simulink model "D_vs_tdc"  (R2018b)
settings: Solver=ode23t  StartTime=0.0  StopTime=model_time  FixedStep=0.0000001  RelTol=1e-3
values from neighbouring files (symbols this model uses):
  config_lambda = [lambda0 lambdainf lambda0l mu v_z]    [vs_ifac_setup_v2.m]
  h = [1 0]'    [setup_compensator_test.m]    (also in vs_ifac_setup_v2.m = 0.003)
  Kp = diag([4   4   4 4 30])    [vs_ifac_setup_v2.m]
  Kv = diag([2    2   2 2 20])    [vs_ifac_setup_v2.m]
  L = 0.003    [vs_ifac_setup_v2.m]
  p0 = cam.plot(P, 'pose', T)    [vs_ifac_setup_v2.m]
  p_des = [412 412 612 612; 412 612 612 412]    [vs_ifac_setup_v2.m]
  q0 = -[3.3, 1.2, -1, 1.75, 6]'    [vs_ifac_setup_v2.m]
undefined symbols (not defined in the file or in its folder): addMass, DiscIntNeverNeededParam, Dnaw, Kaw, Ki, Upaw, variation
libraries: roblocks x15, simulink x1
(part 3 of 3)

== matlab function D_vs_tdc/ARM Plant (MCG)1/C  ==
  data: q input; dq input; tau output
function tau = getC(q, dq)
G3 = 0;

th1 = q(1);
th2 = q(2);
th3 = q(3);
th4 = q(4);
th5 = q(5);

QP1 = dq(1);
QP2 = dq(2);
QP3 = dq(3);
QP4 = dq(4);
QP5 = dq(5);


XX1 = 0;
XY1 = 0;
XZ1 = 0;
YY1 = 0;
YZ1 = 0;
ZZ1 = 0.7569 * 1.0e-04;
MX1 = 0.0165*0.1390;
MY1 = 0;
MZ1 = -0.0300*0.1390;
M1 = 0.1390;
IA1 = 1.3910e-04;

XX2 = 0.0003;
XY2 = 0;
XZ2 = 0;
YY2 = 0.0106;
YZ2 = 0;
ZZ2 = 0.0106;
MX2 = 0.0775*1.3180;
MY2 = 0;
MZ2 = 0;
M2 = 1.3180;
IA2 = 1.3910e-04;

XX3 = 0.0002;
XY3 = 0;
XZ3 = 0;
YY3 = 0.0050;
YZ3 = 0;
ZZ3 = 0.0050;
MX3 = 0.0675*0.8210;
MY3 = 0;
MZ3 = 0;
M3 = 0.8210;
IA3 = 1.3570e-04;

XX4 = 0.0033;
XY4 = 0;
XZ4 = 0;
YY4 = 0.0002;
YZ4 = 0;
ZZ4 = 0.0033;
MX4 = 0;
MY4 = 0.0568*0.7690;
MZ4 = 0;
M4 = 0.7690;
IA4 = 9.3200e-05;

XX5 = 0;
XY5 = 0;
XZ5 = 0;
YY5 = 0;
YZ5 = 0;
ZZ5 = 0.1820 * 1.0e-04;
MX5 = 0;
MY5 = 0;
MZ5 = 0.*0.0910;
M5 = 0.0910;
IA5 = 3.5700e-05;


% Motors parameters
% FS1 = 0.2;
% FV1 = 0.0012;
% FS2 = 0.2;
% FV2 = 0.0012;
% FS3 = 0.2;
% FV3 = 0.0012;
% FS4 = 0.2;
% FV4 =  0.0012;
% FS5 =  0.2;
% FV5 = 0.0012;
% MZ3 = 0.2;

FS1 = 0;
FV1 = 0.0012;
FS2 = 0;
FV2 = 0.0012;
FS3 = 0;
FV3 = 0.0012;
FS4 = 0;
FV4 =  0.0012;
FS5 =  0;
FV5 = 0.0012;



C_th1 = cos(th1 - 2.9496);
S_th1 = sin(th1 - 2.9496);
C_th2 = cos(th2 - 2.7053);
S_th2 = sin(th2 - 2.7053);
S_th3 = sin(th3 + 2.6354);
C_th3 = cos(th3 + 2.6354);
C_th4 = cos(th4 - 3.3598);
S_th4 = sin(th4 - 3.3598);
S_th5 = sin(th5 - 2.8798);
C_th5 = cos(th5 - 2.8798);
DV61 = QP1^2;
W12 = -QP1*S_th2;
W22 = C_th2*QP1;
WP12 = QP2*W22;
WP22 = -QP2*W12;
DV12 = W12^2;
DV22 = W12*W22;
DV42 = W22^2;
DV62 = QP2^2;
U112 = -DV42 - DV62;
U312 = -2*WP22;
U222 = -DV12 - DV62;
U322 = 2*WP12;
U332 = -DV12 - DV42;
VSP12 = -0.033*DV61;
VP12 = C_th2*VSP12 + G3*S_th2;
VP22 = -C_th2*G3 + S_th2*VSP12;
W13 = C_th3*W12 - S_th3*W22;
W23 = C_th3*W22 + S_th3*W12;
W33 = QP2 + QP3;
WP13 = C_th3*WP12 + QP3*W23 - S_th3*WP22;
WP23 = C_th3*WP22 - QP3*W13 + S_th3*WP12;
DV13 = W13^2;
DV23 = W13*W23;
DV33 = W13*W33;
DV43 = W23^2;
DV53 = W23*W33;
DV63 = W33^2;
U113 = -DV43 - DV63;
U313 = DV33 - WP23;
U223 = -DV13 - DV63;
U323 = DV53 + WP13;
U133 = DV33 + WP23;
U233 = DV53 - WP13;
U333 = -DV13 - DV43;
VSP13 = 0.155*U112 + VP12;
VSP23 = 0.155*DV22 + VP22;
VSP33 = 0.155*U312;
VP13 = C_th3*VSP13 - S_th3*VSP23;
VP23 = C_th3*VSP23 + S_th3*VSP13;
W14 = C_th4*W13 - S_th4*W23;
W24 = C_th4*W23 + S_th4*W13;
W34 = QP4 + W33;
WP14 = C_th4*WP13 + QP4*W24 - S_th4*WP23;
WP24 = C_th4*WP23 - QP4*W14 + S_th4*WP13;
DV14 = W14^2;
DV24 = W14*W24;
DV34 = W14*W34;
DV44 = W24^2;
DV54 = W24*W34;
DV64 = W34^2;
U114 = -DV44 - DV64;
U314 = DV34 - WP24;
U224 = -DV14 - DV64;
U324 = DV54 + WP14;
U134 = DV34 + WP24;
U234 = DV54 - WP14;
U334 = -DV14 - DV44;
VSP14 = 0.135*U113 + VP13;
VSP24 = 0.135*DV23 + VP23;
VSP34 = 0.135*U313 + VSP33;
VP14 = C_th4*VSP14 - S_th4*VSP24;
VP24 = C_th4*VSP24 + S_th4*VSP14;
W15 = C_th5*W14 - S_th5*W34;
W25 = C_th5*W34 + S_th5*W14;
W35 = QP5 - W24;
WP15 = C_th5*WP14 + QP5*W25;
WP25 = -QP5*W15 + S_th5*WP14;
DV15 = W15^2;
DV25 = W15*W25;
DV35 = W15*W35;
DV45 = W25^2;
DV55 = W25*W35;
DV65 = W35^2;
U115 = -DV45 - DV65;
U215 = DV25 - WP24;
U315 = DV35 - WP25;
U125 = DV25 + WP24;
U225 = -DV15 - DV65;
U325 = DV55 + WP15;
U135 = DV35 + WP25;
U235 = DV55 - WP15;
U335 = -DV15 - DV45;
VSP15 = -0.218*DV24 + VP14;
VSP25 = -0.218*U224 + VP24;
VSP35 = -0.218*U324 + VSP34;
VP15 = C_th5*VSP15 - S_th5*VSP35;
VP25 = C_th5*VSP35 + S_th5*VSP15;
F11 = -DV61*MX1;
F21 = -DV61*MY1;
F31 = -G3*M1;
PSI11 = QP1*XZ1;
PSI21 = QP1*YZ1;
PSI31 = QP1*ZZ1;
No11 = -PSI21*QP1;
No21 = PSI11*QP1;
F12 = DV22*MY2 + M2*VP12 + MX2*U112;
F22 = DV22*MX2 + M2*VP22 + MY2*U222;
F32 = MX2*U312 + MY2*U322 + MZ2*U332;
PSI12 = QP2*XZ2 + W12*XX2 + W22*XY2;
PSI22 = QP2*YZ2 + W12*XY2 + W22*YY2;
PSI32 = QP2*ZZ2 + W12*XZ2 + W22*YZ2;
No12 = -PSI22*QP2 + PSI32*W22 + WP12*XX2 + WP22*XY2;
No22 = PSI12*QP2 - PSI32*W12 + WP12*XY2 + WP22*YY2;
No32 = -PSI12*W22 + PSI22*W12 + WP12*XZ2 + WP22*YZ2;
F13 = DV23*MY3 + M3*VP13 + MX3*U113 + MZ3*U133;
F23 = DV23*MX3 + M3*VP23 + MY3*U223 + MZ3*U233;
F33 = M3*VSP33 + MX3*U313 + MY3*U323 + MZ3*U333;
PSI13 = W13*XX3 + W23*XY3 + W33*XZ3;
PSI23 = W13*XY3 + W23*YY3 + W33*YZ3;
PSI33 = W13*XZ3 + W23*YZ3 + W33*ZZ3;
No13 = -PSI23*W33 + PSI33*W23 + WP13*XX3 + WP23*XY3;
No23 = PSI13*W33 - PSI33*W13 + WP13*XY3 + WP23*YY3;
No33 = -PSI13*W23 + PSI23*W13 + WP13*XZ3 + WP23*YZ3;
F14 = DV24*MY4 + M4*VP14 + MX4*U114 + MZ4*U134;
F24 = DV24*MX4 + M4*VP24 + MY4*U224 + MZ4*U234;
F34 = M4*VSP34 + MX4*U314 + MY4*U324 + MZ4*U334;
PSI14 = W14*XX4 + W24*XY4 + W34*XZ4;
PSI24 = W14*XY4 + W24*YY4 + W34*YZ4;
PSI34 = W14*XZ4 + W24*YZ4 + W34*ZZ4;
No14 = -PSI24*W34 + PSI34*W24 + WP14*XX4 + WP24*XY4;
No24 = PSI14*W34 - PSI34*W14 + WP14*XY4 + WP24*YY4;
No34 = -PSI14*W24 + PSI24*W14 + WP14*XZ4 + WP24*YZ4;
F15 = M5*VP15 + MX5*U115 + MY5*U125 + MZ5*U135;
F25 = M5*VP25 + MX5*U215 + MY5*U225 + MZ5*U235;
F35 = -M5*VSP25 + MX5*U315 + MY5*U325 + MZ5*U335;
PSI15 = W15*XX5 + W25*XY5 + W35*XZ5;
PSI25 = W15*XY5 + W25*YY5 + W35*YZ5;
PSI35 = W15*XZ5 + W25*YZ5 + W35*ZZ5;
No15 = -PSI25*W35 + PSI35*W25 + WP15*XX5 - WP24*XZ5 + WP25*XY5;
No25 = PSI15*W35 - PSI35*W15 + WP15*XY5 - WP24*YZ5 + WP25*YY5;
No35 = -PSI15*W25 + PSI25*W15 + WP15*XZ5 - WP24*ZZ5 + WP25*YZ5;
N15 = -MY5*VSP25 - MZ5*VP25 + No15;
N25 = MX5*VSP25 + MZ5*VP15 + No25;
N35 = MX5*VP25 - MY5*VP15 + No35;
FDI15 = C_th5*F15 + F25*S_th5;
FDI35 = C_th5*F25 - F15*S_th5;
E14 = F14 + FDI15;
E24 = F24 - F35;
E34 = F34 + FDI35;
N14 = C_th5*N15 - 0.218*FDI35 + MY4*VSP34 - MZ4*VP24 + N25*S_th5 + No14;
N24 = -MX4*VSP34 + MZ4*VP14 - N35 + No24;
N34 = C_th5*N25 + 0.218*FDI15 + MX4*VP24 - MY4*VP14 - N15*S_th5 + No34;
FDI14 = C_th4*E14 + E24*S_th4;
FDI24 = C_th4*E24 - E14*S_th4;
E13 = F13 + FDI14;
E23 = F23 + FDI24;
E33 = E34 + F33;
N13 = C_th4*N14 + MY3*VSP33 - MZ3*VP23 + N24*S_th4 + No13;
N23 = C_th4*N24 - 0.135*E34 - MX3*VSP33 + MZ3*VP13 - N14*S_th4 + No23;
N33 = 0.135*FDI24 + MX3*VP23 - MY3*VP13 + N34 + No33;
FDI13 = C_th3*E13 + E23*S_th3;
FDI23 = C_th3*E23 - E13*S_th3;
E12 = F12 + FDI13;
E22 = F22 + FDI23;
E32 = E33 + F32;
N12 = C_th3*N13 - MZ2*VP22 + N23*S_th3 + No12;
N22 = C_th3*N23 - 0.155*E33 + MZ2*VP12 - N13*S_th3 + No22;
N32 = 0.155*FDI23 + MX2*VP22 - MY2*VP12 + N33 + No32;
FDI12 = C_th2*E12 + E22*S_th2;
FDI32 = C_th2*E22 - E12*S_th2;
E11 = F11 + FDI12;
E21 = -E32 + F21;
E31 = F31 + FDI32;
N11 = C_th2*N12 - G3*MY1 + N22*S_th2 + No11;
N21 = -0.033*FDI32 + G3*MX1 - N32 + No21;
N31 = C_th2*N22 - 0.033*E32 - N12*S_th2;
FDI11 = C_th1*E11 + E21*S_th1;
FDI21 = C_th1*E21 - E11*S_th1;
GAM1 = FS1*sign(QP1) + FV1*QP1 + N31;
GAM2 = FS2*sign(QP2) + FV2*QP2 + N32;
GAM3 = FS3*sign(QP3) + FV3*QP3 + N33;
GAM4 = FS4*sign(QP4) + FV4*QP4 + N34;
GAM5 = FS5*sign(QP5) + FV5*QP5 + N35;

tau = [GAM1 GAM2 GAM3 GAM4 GAM5]';

== matlab function D_vs_tdc/MCG (Symoro, DD)/C  ==
  data: q input; dq input; tau output
function tau = getC(q, dq)
G3 = -9.81;

th1 = q(1);
th2 = q(2);
th3 = q(3);
th4 = q(4);
th5 = q(5);

QP1 = dq(1);
QP2 = dq(2);
QP3 = dq(3);
QP4 = dq(4);
QP5 = dq(5);


XX1 = 0;
XY1 = 0;
XZ1 = 0;
YY1 = 0;
YZ1 = 0;
ZZ1 = 0.7569 * 1.0e-04;
MX1 = 0.0165*0.1390;
MY1 = 0;
MZ1 = -0.0300;
M1 = 0.1390;
IA1 = 1.3910e-04;

XX2 = 0.0003;
XY2 = 0;
XZ2 = 0;
YY2 = 0.0106;
YZ2 = 0;
ZZ2 = 0.0106;
MX2 = 0.0775*1.3180;
MY2 = 0;
MZ2 = 0;
M2 = 1.3180;
IA2 = 1.3910e-04;

XX3 = 0.0002;
XY3 = 0;
XZ3 = 0;
YY3 = 0.0050;
YZ3 = 0;
ZZ3 = 0.0050;
MX3 = 0.0675*0.8210;
MY3 = 0;
MZ3 = 0;
M3 = 0.8210;
IA3 = 1.3570e-04;

XX4 = 0.0033;
XY4 = 0;
XZ4 = 0;
YY4 = 0.0002;
YZ4 = 0;
ZZ4 = 0.0033;
MX4 = 0;
MY4 = 0.0568*0.7690;
MZ4 = 0;
M4 = 0.7690;
IA4 = 9.3200e-05;

XX5 = 0;
XY5 = 0;
XZ5 = 0;
YY5 = 0;
YZ5 = 0;
ZZ5 = 0.1820 * 1.0e-04;
MX5 = 0;
MY5 = 0;
MZ5 = 0.*0.0910;
M5 = 0.0910;
IA5 = 3.5700e-05;


% Motors parameters
FS1 = 0;
FV1 = 0.0012;
FS2 = 0;
FV2 = 0.0012;
FS3 = 0;
FV3 = 0.0012;
FS4 = 0;
FV4 =  0.0012;
FS5 = 0;
FV5 = 0.0012;

% FS1 = 0;
% FV1 = 0;
% FS2 = 0;
% FV2 = 0;
% FS3 = 0;
% FV3 = 0;
% FS4 = 0;
% FV4 = 0;
% FS5 = 0;
% FV5 = 0;


C_th1 = cos(th1 - 2.9496);
S_th1 = sin(th1 - 2.9496);
C_th2 = cos(th2 - 2.7053);
S_th2 = sin(th2 - 2.7053);
S_th3 = sin(th3 + 2.6354);
C_th3 = cos(th3 + 2.6354);
C_th4 = cos(th4 - 3.3598);
S_th4 = sin(th4 - 3.3598);
S_th5 = sin(th5 - 2.8798);
C_th5 = cos(th5 - 2.8798);
DV61 = QP1^2;
W12 = -QP1*S_th2;
W22 = C_th2*QP1;
WP12 = QP2*W22;
WP22 = -QP2*W12;
DV12 = W12^2;
DV22 = W12*W22;
DV42 = W22^2;
DV62 = QP2^2;
U112 = -DV42 - DV62;
U312 = -2*WP22;
U222 = -DV12 - DV62;
U322 = 2*WP12;
U332 = -DV12 - DV42;
VSP12 = -0.033*DV61;
VP12 = C_th2*VSP12 + G3*S_th2;
VP22 = -C_th2*G3 + S_th2*VSP12;
W13 = C_th3*W12 - S_th3*W22;
W23 = C_th3*W22 + S_th3*W12;
W33 = QP2 + QP3;
WP13 = C_th3*WP12 + QP3*W23 - S_th3*WP22;
WP23 = C_th3*WP22 - QP3*W13 + S_th3*WP12;
DV13 = W13^2;
DV23 = W13*W23;
DV33 = W13*W33;
DV43 = W23^2;
DV53 = W23*W33;
DV63 = W33^2;
U113 = -DV43 - DV63;
U313 = DV33 - WP23;
U223 = -DV13 - DV63;
U323 = DV53 + WP13;
U133 = DV33 + WP23;
U233 = DV53 - WP13;
U333 = -DV13 - DV43;
VSP13 = 0.155*U112 + VP12;
VSP23 = 0.155*DV22 + VP22;
VSP33 = 0.155*U312;
VP13 = C_th3*VSP13 - S_th3*VSP23;
VP23 = C_th3*VSP23 + S_th3*VSP13;
W14 = C_th4*W13 - S_th4*W23;
W24 = C_th4*W23 + S_th4*W13;
W34 = QP4 + W33;
WP14 = C_th4*WP13 + QP4*W24 - S_th4*WP23;
WP24 = C_th4*WP23 - QP4*W14 + S_th4*WP13;
DV14 = W14^2;
DV24 = W14*W24;
DV34 = W14*W34;
DV44 = W24^2;
DV54 = W24*W34;
DV64 = W34^2;
U114 = -DV44 - DV64;
U314 = DV34 - WP24;
U224 = -DV14 - DV64;
U324 = DV54 + WP14;
U134 = DV34 + WP24;
U234 = DV54 - WP14;
U334 = -DV14 - DV44;
VSP14 = 0.135*U113 + VP13;
VSP24 = 0.135*DV23 + VP23;
VSP34 = 0.135*U313 + VSP33;
VP14 = C_th4*VSP14 - S_th4*VSP24;
VP24 = C_th4*VSP24 + S_th4*VSP14;
W15 = C_th5*W14 - S_th5*W34;
W25 = C_th5*W34 + S_th5*W14;
W35 = QP5 - W24;
WP15 = C_th5*WP14 + QP5*W25;
WP25 = -QP5*W15 + S_th5*WP14;
DV15 = W15^2;
DV25 = W15*W25;
DV35 = W15*W35;
DV45 = W25^2;
DV55 = W25*W35;
DV65 = W35^2;
U115 = -DV45 - DV65;
U215 = DV25 - WP24;
U315 = DV35 - WP25;
U125 = DV25 + WP24;
U225 = -DV15 - DV65;
U325 = DV55 + WP15;
U135 = DV35 + WP25;
U235 = DV55 - WP15;
U335 = -DV15 - DV45;
VSP15 = -0.218*DV24 + VP14;
VSP25 = -0.218*U224 + VP24;
VSP35 = -0.218*U324 + VSP34;
VP15 = C_th5*VSP15 - S_th5*VSP35;
VP25 = C_th5*VSP35 + S_th5*VSP15;
F11 = -DV61*MX1;
F21 = -DV61*MY1;
F31 = -G3*M1;
PSI11 = QP1*XZ1;
PSI21 = QP1*YZ1;
PSI31 = QP1*ZZ1;
No11 = -PSI21*QP1;
No21 = PSI11*QP1;
F12 = DV22*MY2 + M2*VP12 + MX2*U112;
F22 = DV22*MX2 + M2*VP22 + MY2*U222;
F32 = MX2*U312 + MY2*U322 + MZ2*U332;
PSI12 = QP2*XZ2 + W12*XX2 + W22*XY2;
PSI22 = QP2*YZ2 + W12*XY2 + W22*YY2;
PSI32 = QP2*ZZ2 + W12*XZ2 + W22*YZ2;
No12 = -PSI22*QP2 + PSI32*W22 + WP12*XX2 + WP22*XY2;
No22 = PSI12*QP2 - PSI32*W12 + WP12*XY2 + WP22*YY2;
No32 = -PSI12*W22 + PSI22*W12 + WP12*XZ2 + WP22*YZ2;
F13 = DV23*MY3 + M3*VP13 + MX3*U113 + MZ3*U133;
F23 = DV23*MX3 + M3*VP23 + MY3*U223 + MZ3*U233;
F33 = M3*VSP33 + MX3*U313 + MY3*U323 + MZ3*U333;
PSI13 = W13*XX3 + W23*XY3 + W33*XZ3;
PSI23 = W13*XY3 + W23*YY3 + W33*YZ3;
PSI33 = W13*XZ3 + W23*YZ3 + W33*ZZ3;
No13 = -PSI23*W33 + PSI33*W23 + WP13*XX3 + WP23*XY3;
No23 = PSI13*W33 - PSI33*W13 + WP13*XY3 + WP23*YY3;
No33 = -PSI13*W23 + PSI23*W13 + WP13*XZ3 + WP23*YZ3;
F14 = DV24*MY4 + M4*VP14 + MX4*U114 + MZ4*U134;
F24 = DV24*MX4 + M4*VP24 + MY4*U224 + MZ4*U234;
F34 = M4*VSP34 + MX4*U314 + MY4*U324 + MZ4*U334;
PSI14 = W14*XX4 + W24*XY4 + W34*XZ4;
PSI24 = W14*XY4 + W24*YY4 + W34*YZ4;
PSI34 = W14*XZ4 + W24*YZ4 + W34*ZZ4;
No14 = -PSI24*W34 + PSI34*W24 + WP14*XX4 + WP24*XY4;
No24 = PSI14*W34 - PSI34*W14 + WP14*XY4 + WP24*YY4;
No34 = -PSI14*W24 + PSI24*W14 + WP14*XZ4 + WP24*YZ4;
F15 = M5*VP15 + MX5*U115 + MY5*U125 + MZ5*U135;
F25 = M5*VP25 + MX5*U215 + MY5*U225 + MZ5*U235;
F35 = -M5*VSP25 + MX5*U315 + MY5*U325 + MZ5*U335;
PSI15 = W15*XX5 + W25*XY5 + W35*XZ5;
PSI25 = W15*XY5 + W25*YY5 + W35*YZ5;
PSI35 = W15*XZ5 + W25*YZ5 + W35*ZZ5;
No15 = -PSI25*W35 + PSI35*W25 + WP15*XX5 - WP24*XZ5 + WP25*XY5;
No25 = PSI15*W35 - PSI35*W15 + WP15*XY5 - WP24*YZ5 + WP25*YY5;
No35 = -PSI15*W25 + PSI25*W15 + WP15*XZ5 - WP24*ZZ5 + WP25*YZ5;
N15 = -MY5*VSP25 - MZ5*VP25 + No15;
N25 = MX5*VSP25 + MZ5*VP15 + No25;
N35 = MX5*VP25 - MY5*VP15 + No35;
FDI15 = C_th5*F15 + F25*S_th5;
FDI35 = C_th5*F25 - F15*S_th5;
E14 = F14 + FDI15;
E24 = F24 - F35;
E34 = F34 + FDI35;
N14 = C_th5*N15 - 0.218*FDI35 + MY4*VSP34 - MZ4*VP24 + N25*S_th5 + No14;
N24 = -MX4*VSP34 + MZ4*VP14 - N35 + No24;
N34 = C_th5*N25 + 0.218*FDI15 + MX4*VP24 - MY4*VP14 - N15*S_th5 + No34;
FDI14 = C_th4*E14 + E24*S_th4;
FDI24 = C_th4*E24 - E14*S_th4;
E13 = F13 + FDI14;
E23 = F23 + FDI24;
E33 = E34 + F33;
N13 = C_th4*N14 + MY3*VSP33 - MZ3*VP23 + N24*S_th4 + No13;
N23 = C_th4*N24 - 0.135*E34 - MX3*VSP33 + MZ3*VP13 - N14*S_th4 + No23;
N33 = 0.135*FDI24 + MX3*VP23 - MY3*VP13 + N34 + No33;
FDI13 = C_th3*E13 + E23*S_th3;
FDI23 = C_th3*E23 - E13*S_th3;
E12 = F12 + FDI13;
E22 = F22 + FDI23;
E32 = E33 + F32;
N12 = C_th3*N13 - MZ2*VP22 + N23*S_th3 + No12;
N22 = C_th3*N23 - 0.155*E33 + MZ2*VP12 - N13*S_th3 + No22;
N32 = 0.155*FDI23 + MX2*VP22 - MY2*VP12 + N33 + No32;
FDI12 = C_th2*E12 + E22*S_th2;
FDI32 = C_th2*E22 - E12*S_th2;
E11 = F11 + FDI12;
E21 = -E32 + F21;
E31 = F31 + FDI32;
N11 = C_th2*N12 - G3*MY1 + N22*S_th2 + No11;
N21 = -0.033*FDI32 + G3*MX1 - N32 + No21;
N31 = C_th2*N22 - 0.033*E32 - N12*S_th2;
FDI11 = C_th1*E11 + E21*S_th1;
FDI21 = C_th1*E21 - E11*S_th1;
GAM1 = FS1*sign(QP1) + FV1*QP1 + N31;
GAM2 = FS2*sign(QP2) + FV2*QP2 + N32;
GAM3 = FS3*sign(QP3) + FV3*QP3 + N33;
GAM4 = FS4*sign(QP4) + FV4*QP4 + N34;
GAM5 = FS5*sign(QP5) + FV5*QP5 + N35;

tau = [GAM1 GAM2 GAM3 GAM4 GAM5]';

== matlab function D_vs_tdc/MCG (Symoro, DD)/M (Symoro) ==
  data: q input; A output
function A = fcn(q)
G3 = -9.81;

th1 = q(1);
th2 = q(2);
th3 = q(3);
th4 = q(4);
th5 = q(5);

XX1 = 0;
XY1 = 0;
XZ1 = 0;
YY1 = 0;
YZ1 = 0;
ZZ1 = 0.7569 * 1.0e-04;
MX1 = 0.0165;
MY1 = 0;
MZ1 = -0.0300;
M1 = 0.1390;
IA1 = 1.3910e-04;

XX2 = 0.0003;
XY2 = 0;
XZ2 = 0;
YY2 = 0.0106;
YZ2 = 0;
ZZ2 = 0.0106;
MX2 = 0.0775*1.3180;
MY2 = 0;
MZ2 = 0;
M2 = 1.3180;
IA2 = 1.3910e-04;

XX3 = 0.0002;
XY3 = 0;
XZ3 = 0;
YY3 = 0.0050;
YZ3 = 0;
ZZ3 = 0.0050;
MX3 = 0.0675*0.8210;
MY3 = 0;
MZ3 = 0;
M3 = 0.8210;
IA3 = 1.3570e-04;

XX4 = 0.0033;
XY4 = 0;
XZ4 = 0;
YY4 = 0.0002;
YZ4 = 0;
ZZ4 = 0.0033;
MX4 = 0;
MY4 = 0.0568*0.7690;
MZ4 = 0;
M4 = 0.7690;
IA4 = 9.3200e-05;

XX5 = 0;FS1 = 10;
FV1 = 0.0012*100;
FS2 = 10;
FV2 = 0.0012*100;
FS3 = 10;
FV3 = 0.0012*100;
FS4 = 10;
FV4 =  0.0012*100;
FS5 = 10;
FV5 = 0.0012*100;
XY5 = 0;
XZ5 = 0;
YY5 = 0;
YZ5 = 0;
ZZ5 = 0.1820 * 1.0e-04;
MX5 = 0;
MY5 = 0;
MZ5 = 0.*0.0910;
M5 = 0.0910;
IA5 = 3.5700e-05;


% Motors parameters
FS1 = 0;
FV1 = 0.0012;
FS2 = 0;
FV2 = 0.0012;
FS3 = 0;
FV3 = 0.0012;
FS4 = 0;
FV4 =  0.0012;
FS5 = 0;
FV5 = 0.0012;

% FS1 = 0;
% FV1 = 0;
% FS2 = 0;
% FV2 = 0;
% FS3 = 0;
% FV3 = 0;
% FS4 = 0;
% FV4 = 0;
% FS5 = 0;
% FV5 = 0;


C_th1 = cos(th1 - 2.9496);
S_th1 = sin(th1 - 2.9496);
C_th2 = cos(th2 - 2.7053);
S_th2 = sin(th2 - 2.7053);
S_th3 = sin(th3 + 2.6354);
C_th3 = cos(th3 + 2.6354);
C_th4 = cos(th4 - 3.3598);
S_th4 = sin(th4 - 3.3598);
S_th5 = sin(th5 - 2.8798);
C_th5 = cos(th5 - 2.8798);
AS15 = C_th5*MX5 + MY5*S_th5;
AS35 = C_th5*MY5 - MX5*S_th5;
AJ115 = C_th5*XX5 + S_th5*XY5;
AJ315 = C_th5*XY5 - S_th5*XX5;
AJ125 = C_th5*XY5 + S_th5*YY5;
AJ325 = C_th5*YY5 - S_th5*XY5;
AJ135 = C_th5*XZ5 + S_th5*YZ5;
AJ335 = C_th5*YZ5 - S_th5*XZ5;
AJA115 = AJ115*C_th5 + AJ125*S_th5;
AJA315 = AJ315*C_th5 + AJ325*S_th5;
AJA135 = -AJ115*S_th5 + AJ125*C_th5;
AJA335 = -AJ315*S_th5 + AJ325*C_th5;
PAS115 = -0.218*MZ5;
PAS125 = -0.218*AS15;
PAS325 = -0.218*AS35;
JP114 = AJA115 + 0.047524*M5 - 2*PAS115 + XX4;
JP214 = -AJ135 - PAS125 + XY4;
JP314 = AJA315 + XZ4;
JP224 = YY4 + ZZ5;
JP324 = -AJ335 - PAS325 + YZ4;
JP134 = AJA135 + XZ4;
JP334 = AJA335 + 0.047524*M5 - 2*PAS115 + ZZ4;
MSP14 = AS15 + MX4;
MSP24 = -0.218*M5 + MY4 - MZ5;
MSP34 = AS35 + MZ4;
MP4 = M4 + M5;
AS14 = C_th4*MSP14 + MSP24*S_th4;
AS24 = C_th4*MSP24 - MSP14*S_th4;
AJ114 = C_th4*JP114 + JP214*S_th4;
AJ214 = C_th4*JP214 - JP114*S_th4;
AJ124 = C_th4*JP214 + JP224*S_th4;
AJ224 = C_th4*JP224 - JP214*S_th4;
AJ134 = C_th4*JP134 + JP324*S_th4;
AJ234 = C_th4*JP324 - JP134*S_th4;
AJA114 = AJ114*C_th4 + AJ124*S_th4;
AJA214 = AJ214*C_th4 + AJ224*S_th4;
AJA314 = C_th4*JP314 + JP324*S_th4;
AJA124 = -AJ114*S_th4 + AJ124*C_th4;
AJA224 = -AJ214*S_th4 + AJ224*C_th4;
AJA324 = C_th4*JP324 - JP314*S_th4;
PAS214 = 0.135*AS24;
PAS314 = 0.135*MSP34;
PAS224 = -0.135*AS14;
JP113 = AJA114 + XX3;
JP213 = AJA214 - PAS214 + XY3;
JP313 = AJA314 - PAS314 + XZ3;
JP123 = AJA124 - PAS214 + XY3;
JP223 = AJA224 + 0.018225*MP4 - 2*PAS224 + YY3;
JP323 = AJA324 + YZ3;
JP133 = AJ134 - PAS314 + XZ3;
JP233 = AJ234 + YZ3;
JP333 = JP334 + 0.018225*MP4 - 2*PAS224 + ZZ3;
MSP13 = AS14 + 0.135*MP4 + MX3;
MSP23 = AS24 + MY3;
MSP33 = MSP34 + MZ3;
MP3 = M3 + MP4;
AS13 = C_th3*MSP13 + MSP23*S_th3;
AS23 = C_th3*MSP23 - MSP13*S_th3;
AJ113 = C_th3*JP113 + JP213*S_th3;
AJ213 = C_th3*JP213 - JP113*S_th3;
AJ123 = C_th3*JP123 + JP223*S_th3;
AJ223 = C_th3*JP223 - JP123*S_th3;
AJ133 = C_th3*JP133 + JP233*S_th3;
AJ233 = C_th3*JP233 - JP133*S_th3;
AJA113 = AJ113*C_th3 + AJ123*S_th3;
AJA213 = AJ213*C_th3 + AJ223*S_th3;
AJA313 = C_th3*JP313 + JP323*S_th3;
AJA123 = -AJ113*S_th3 + AJ123*C_th3;
AJA223 = -AJ213*S_th3 + AJ223*C_th3;
AJA323 = C_th3*JP323 - JP313*S_th3;
PAS213 = 0.155*AS23;
PAS313 = 0.155*MSP33;
PAS223 = -0.155*AS13;
JP112 = AJA113 + XX2;
JP212 = AJA213 - PAS213 + XY2;
JP312 = AJA313 - PAS313 + XZ2;
JP122 = AJA123 - PAS213 + XY2;
JP222 = AJA223 + 0.024025*MP3 - 2*PAS223 + YY2;
JP322 = AJA323 + YZ2;
JP132 = AJ133 - PAS313 + XZ2;
JP232 = AJ233 + YZ2;
JP332 = JP333 + 0.024025*MP3 - 2*PAS223 + ZZ2;
MSP12 = AS13 + 0.155*MP3 + MX2;
MSP22 = AS23 + MY2;
MSP32 = MSP33 + MZ2;
MP2 = M2 + MP3;
AS12 = C_th2*MSP12 + MSP22*S_th2;
AS32 = C_th2*MSP22 - MSP12*S_th2;
AJ112 = C_th2*JP112 + JP212*S_th2;
AJ312 = C_th2*JP212 - JP112*S_th2;
AJ122 = C_th2*JP122 + JP222*S_th2;
AJ322 = C_th2*JP222 - JP122*S_th2;
AJ132 = C_th2*JP132 + JP232*S_th2;
AJ332 = C_th2*JP232 - JP132*S_th2;
AJA112 = AJ112*C_th2 + AJ122*S_th2;
AJA212 = -C_th2*JP312 - JP322*S_th2;
AJA312 = AJ312*C_th2 + AJ322*S_th2;
AJA132 = -AJ112*S_th2 + AJ122*C_th2;
AJA232 = -C_th2*JP322 + JP312*S_th2;
AJA332 = -AJ312*S_th2 + AJ322*C_th2;
PAS212 = -0.033*MSP32;
PAS312 = 0.033*AS32;
PAS222 = -0.033*AS12;
JP111 = AJA112 + XX1;
JP211 = AJA212 - PAS212 + XY1;
JP311 = AJA312 - PAS312 + XZ1;
JP121 = -AJ132 - PAS212 + XY1;
JP221 = JP332 + 0.001089*MP2 - 2*PAS222 + YY1;
JP321 = -AJ332 + YZ1;
JP131 = AJA132 - PAS312 + XZ1;
JP231 = AJA232 + YZ1;
JP331 = AJA332 + 0.001089*MP2 - 2*PAS222 + ZZ1;
MSP11 = AS12 + 0.033*MP2 + MX1;
MSP21 = -MSP32 + MY1;
MSP31 = AS32 + MZ1;
MP1 = M1 + MP2;
Nc21 = -0.033*C_th2*MSP12 - JP332 - 0.033*MSP22*S_th2;
Nd32 = 0.155*C_th3*MSP13 + JP333 + 0.155*MSP23*S_th3;
Ed11 = AS13*S_th2 - AS23*C_th2;
Ed31 = AS13*C_th2 + AS23*S_th2;
Nd11 = AJ133*C_th2 + AJ233*S_th2;
Nd21 = -0.033*AS13*C_th2 - 0.033*AS23*S_th2 - Nd32;
Nd31 = -AJ133*S_th2 + AJ233*C_th2;
Ne33 = 0.135*C_th4*MSP14 + JP334 + 0.135*MSP24*S_th4;
Ee12 = AS14*S_th3 - AS24*C_th3;
Ee22 = AS14*C_th3 + AS24*S_th3;
Ne12 = AJ134*C_th3 + AJ234*S_th3;
Ne22 = -AJ134*S_th3 + AJ234*C_th3;
Ne32 = 0.155*AS14*C_th3 + 0.155*AS24*S_th3 + Ne33;
Ee11 = C_th2*Ee12 + Ee22*S_th2;
Ee31 = C_th2*Ee22 - Ee12*S_th2;
Ne11 = C_th2*Ne12 + Ne22*S_th2;
Ne21 = -0.033*C_th2*Ee22 + 0.033*Ee12*S_th2 - Ne32;
Ne31 = C_th2*Ne22 - Ne12*S_th2;
Nf14 = AJ135 - 0.218*C_th5*MX5 - 0.218*MY5*S_th5;
Nf34 = AJ335 - 0.218*C_th5*MY5 + 0.218*MX5*S_th5;
Ef13 = -AS35*C_th4;
Ef23 = AS35*S_th4;
Nf13 = C_th4*Nf14 - S_th4*ZZ5;
Nf23 = -0.135*AS15 - C_th4*ZZ5 - Nf14*S_th4;
Nf33 = 0.135*AS35*S_th4 + Nf34;
Ef12 = C_th3*Ef13 + Ef23*S_th3;
Ef22 = C_th3*Ef23 - Ef13*S_th3;
Nf12 = C_th3*Nf13 + Nf23*S_th3;
Nf22 = -0.155*AS15 + C_th3*Nf23 - Nf13*S_th3;
Nf32 = 0.155*C_th3*Ef23 - 0.155*Ef13*S_th3 + Nf33;
Ef11 = C_th2*Ef12 + Ef22*S_th2;
Ef31 = C_th2*Ef22 - Ef12*S_th2;
Nf11 = C_th2*Nf12 + Nf22*S_th2;
Nf21 = -0.033*C_th2*Ef22 + 0.033*Ef12*S_th2 - Nf32;
Nf31 = -0.033*AS15 + C_th2*Nf22 - Nf12*S_th2;
A11 = IA1 + JP331;
A21 = AJ332;
A31 = Nd31;
A41 = Ne31;
A51 = Nf31;
A22 = IA2 + JP332;
A32 = Nd32;
A42 = Ne32;
A52 = Nf32;
A33 = IA3 + JP333;
A43 = Ne33;
A53 = Nf33;
A44 = IA4 + JP334;
A54 = Nf34;
A55 = IA5 + ZZ5;

A = zeros(5,5);
A(1,1) = A11;
A(2,1) = A21;
A(3,1) = A31;
A(4,1) = A41;
A(5,1) = A51;

A(2,2) = A22;
A(3,2) = A32;
A(4,2) = A42;
A(5,2) = A52;

A(3,3) = A33;
A(4,3) = A43;
A(5,3) = A53;

A(4,4) = A44;
A(5,4) = A54;

A(5,5) = A55;

%A = A; %' * inv(A*A' + 0.001 * eye(5,5));

== matlab function D_vs_tdc/MCG (Symoro, DD)/gravity only ==
  data: q input; tau output
function tau = getDfull(q)
G3 = -9.81;
    
th2 = q(2);
th3 = q(3);
th4 = q(4);
th5 = q(5);

C_th2 = cos(th2 - 2.7053);
S_th2 = sin(th2 - 2.7053);
S_th3 = sin(th3 + 2.6354);
C_th3 = cos(th3 + 2.6354);
C_th4 = cos(th4 - 3.3598);
S_th4 = sin(th4 - 3.3598);
S_th5 = sin(th5 - 2.8798);
C_th5 = cos(th5 - 2.8798);


VP12 = G3*S_th2;
VP22 = -C_th2*G3;
VSP13 = VP12;
VSP23 = VP22;
VP13 = C_th3*VSP13 - S_th3*VSP23;
VP23 = C_th3*VSP23 + S_th3*VSP13;
VSP14 = VP13;
VSP24 = VP23;
VP14 = C_th4*VSP14 - S_th4*VSP24;
VP24 = C_th4*VSP24 + S_th4*VSP14;
VSP15 =  VP14;
VSP25 =  VP24;
VP15 = C_th5*VSP15;
VP25 = S_th5*VSP15;
DG2MX2 = VP22;
DG2MY2 = -VP12;
N23MX3 = VP23;
DG2MX3 = N23MX3;C_th2 = cos(th2 - 2.7053);
S_th2 = sin(th2 - 2.7053);
S_th3 = sin(th3 + 2.6354);
C_th3 = cos(th3 + 2.6354);
C_th4 = cos(th4 - 3.3598);
S_th4 = sin(th4 - 3.3598);
S_th5 = sin(th5 - 2.8798);
C_th5 = cos(th5 - 2.8798);
DG3MX3 = VP23;
N23MY3 = - VP13;
DG2MY3 = N23MY3;
DG3MY3 = -VP13;
N33MX4 = VP24;
N23MX4 =  N33MX4;
DG2MX4 = N23MX4;
DG3MX4 = N33MX4;
DG4MX4 = VP24;
N33MY4 = - VP14;
N23MY4 =  N33MY4;
DG2MY4 = N23MY4;
DG3MY4 = N33MY4;
DG4MY4 = -VP14;
N41MX5 = S_th5*VSP25;
N43MX5 = C_th5*VSP25;
N31MX5 = C_th4*N41MX5 - S_th4*VP25;
N32MX5 = -C_th4*VP25 - N41MX5*S_th4;
N33MX5 = N43MX5;
N21MX5 = C_th3*N31MX5 + N32MX5*S_th3;
N22MX5 = C_th3*N32MX5 - N31MX5*S_th3;
N23MX5 = N33MX5;
N13MX5 = C_th2*N22MX5 - N21MX5*S_th2;
DG1MX5 = N13MX5;
DG2MX5 = N23MX5;
DG3MX5 = N33MX5;
DG4MX5 = N43MX5;
DG5MX5 = VP25;
N41MY5 = -C_th5*VSP25;
N43MY5 = S_th5*VSP25;
N31MY5 = C_th4*N41MY5 + S_th4*VP15;
N32MY5 = C_th4*VP15 - N41MY5*S_th4;
N33MY5 = N43MY5;
FDI32MY5 = - 0*S_th3;
N21MY5 = C_th3*N31MY5 + N32MY5*S_th3;
N22MY5 = C_th3*N32MY5 - N31MY5*S_th3;
N23MY5 = 0.155*FDI32MY5 + N33MY5;
N13MY5 = C_th2*N22MY5 - N21MY5*S_th2;
DG1MY5 = N13MY5;
DG2MY5 = N23MY5;
DG3MY5 = N33MY5;
DG4MY5 = N43MY5;
DG5MY5 = -VP15;


%%%%%%%%%%%%%%%%%%%
%%%%%%%%%%%%%%%%%%%%%%%%%%%%%%%%%%%%%%
%%%%%%%%%%%%%%%%%%%%%%%%%%%%%%%%%%%%%%%%%%%%%%%%%%%%%%%%%

MX2 = 0.0775*1.3180;
MY2 = 0;

MX3 = 0.0675*0.8210;
MY3 = 0;
M3 = 0.8210;

MX4 = 0;
MY4 = 0.0568*0.7690;
M4 = 0.7690;

MX5 = 0;
MY5 = 0;
MZ5 = 0.*0.0910;
M5 = 0.0910;


MR4 = M4 + M5;
MYR4 = -0.1136*M5 + MY4 - MZ5;
MR3 = M3 + MR4;
MXR3 = 0.135*MR4 + MX3;
MXR2 = 0.155*MR3 + MX2;



chi = [MXR2 0 MXR3 MY3 MX4 MYR4 MX5 MY5];

D = [
    0,0,0,0,0,0,DG1MX5,DG1MY5;
    DG2MX2,DG2MY2,DG2MX3,DG2MY3,DG2MX4,DG2MY4,DG2MX5,DG2MY5;
    0,0,          DG3MX3,DG3MY3,DG3MX4,DG3MY4,DG3MX5,DG3MY5;
    0,0, 0,0,                   DG4MX4,DG4MY4,DG4MX5,DG4MY5;
    0,0, 0,0, 0,0,                            DG5MX5,DG5MY5
];


tau = D * chi';
